simulink model "sampleModel7127"  (R2017a)
settings: Solver=VariableStepAuto  StartTime=0.0  StopTime=10.0  RelTol=1e-3
undefined symbols (not defined in the file or in its folder): DiscIntNeverNeededParam, sigbuilder_block
libraries: simulink x258
(part 1 of 4)
settings Model: Creator=cyfuzz  LastModifiedBy=cyfuzz

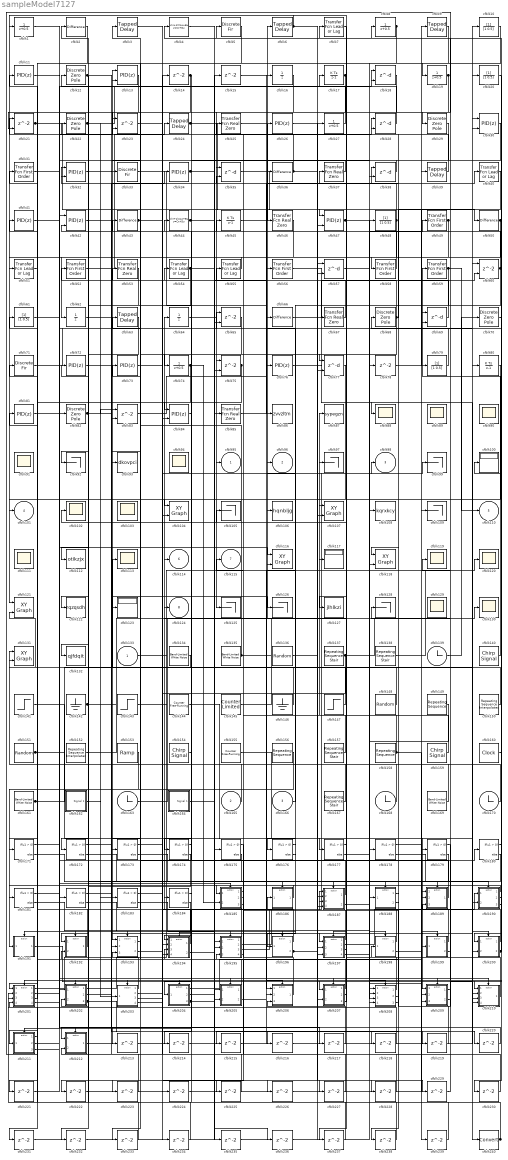
== system sampleModel7127 ==
  cfblk133 : Inport
  cfblk165 : Inport  Port=2
  cfblk166 : Inport  Port=3
  cfblk{1,8,19,27,74} (5 alike) : DiscreteTransferFcn  SampleTime=1
  cfblk{10,20,48,61,79} (5 alike) : DiscreteFilter  SampleTime=1
  cfblk100 : Display
  cfblk{88..91,94,102..103,111,113,119..120,129..130} (13 alike) : Scope
      cfblk103 settings: Floating=on
      cfblk111 settings: Floating=on
      cfblk129 settings: Floating=on
      cfblk89 settings: Floating=on
      cfblk90 settings: Floating=on
      cfblk91 settings: Floating=on
      cfblk94 settings: Floating=on
  cfblk{104,107,116,118,121,131} (6 alike) : simulink/Sinks/XY Graph  xmin=-1  xmax=1  ymin=-1  ymax=1  st=-1
  cfblk{92,97,99,105,109,125..126,128} (8 alike) : Terminator
  cfblk106 : ToWorkspace  VariableName=hqnbljg  SaveFormat=Timeseries  SampleTime=-1
  cfblk108 : ToWorkspace  VariableName=kqrxkcy  SaveFormat=Timeseries  SampleTime=-1
  cfblk{11,26,34,41,72..73,76,81} (8 alike) : simulink/Continuous/PID Controller  Controller=PID  TimeDomain=Discrete-time  SampleTime=1  IntegratorMethod=Forward Euler  FilterMethod=Forward Euler  Form=Parallel  UseFilter=on  ControllerParametersSource=internal  P=1  I=1  D=0  N=100  InitialConditionSource=internal  InitialConditionForIntegrator=0  InitialConditionForFilter=0  ExternalReset=none  LimitOutput=off  UpperSaturationLimit=inf  LowerSaturationLimit=-inf  LinearizeAsGain=off  AntiWindupMode=none  Kb=1  TrackingMode=off  Kt=1  PParamMin=[]  PParamMax=[]  IParamMin=[]  IParamMax=[]  DParamMin=[]  DParamMax=[]  NParamMin=[]  NParamMax=[]  KbParamMin=[]  KbParamMax=[]  KtParamMin=[]  KtParamMax=[]  POutMin=[]  POutMax=[]  IOutMin=[]  IOutMax=[]  DOutMin=[]  DOutMax=[]  NOutMin=[]  NOutMax=[]  KbOutMin=[]  KbOutMax=[]  KtOutMin=[]  KtOutMax=[]  IntegratorOutMin=[]  IntegratorOutMax=[]  FilterOutMin=[]  FilterOutMax=[]  SumOutMin=[]  SumOutMax=[]  SumI1OutMin=[]  SumI1OutMax=[]  SumI2OutMin=[]  SumI2OutMax=[]  SumI3OutMin=[]  SumI3OutMax=[]  SumDOutMin=[]  SumDOutMax=[]  SaturationOutMin=[]  SaturationOutMax=[]  IntegratorContinuousStateAttributes=''  IntegratorStateMustResolveToSignalObject=off  IntegratorRTWStateStorageClass=Auto  FilterContinuousStateAttributes=''  FilterStateMustResolveToSignalObject=off  FilterRTWStateStorageClass=Auto  DifferentiatorICPrevScaledInput=0  DifferentiatorOutMin=[]  DifferentiatorOutMax=[]  InitialConditionSetting=State (most efficient)
  cfblk112 : ToWorkspace  VariableName=otikzjx  SaveFormat=Timeseries  SampleTime=-1
  cfblk117 : Display
  cfblk{12,22,29,68,70,82} (6 alike) : DiscreteZeroPole  Poles=[0 0.5]  Gain=1
  cfblk122 : ToWorkspace  VariableName=rqzqsdh  SaveFormat=Timeseries  SampleTime=-1
  cfblk123 : Display
  cfblk127 : ToWorkspace  VariableName=jlhlkzi  SaveFormat=Timeseries  SampleTime=-1
  cfblk{13,30,32,42,47,84} (6 alike) : simulink/Continuous/PID Controller (2DOF)  Controller=PID  TimeDomain=Discrete-time  SampleTime=1  IntegratorMethod=Forward Euler  FilterMethod=Forward Euler  Form=Parallel  UseFilter=on  ControllerParametersSource=internal  P=1  I=1  D=0  N=100  b=1  c=1  InitialConditionSource=internal  InitialConditionForIntegrator=0  InitialConditionForFilter=0  ExternalReset=none  LimitOutput=off  UpperSaturationLimit=inf  LowerSaturationLimit=-inf  LinearizeAsGain=off  AntiWindupMode=none  Kb=1  TrackingMode=off  Kt=1  PParamMin=[]  PParamMax=[]  IParamMin=[]  IParamMax=[]  DParamMin=[]  DParamMax=[]  NParamMin=[]  NParamMax=[]  bParamMin=[]  bParamMax=[]  cParamMin=[]  cParamMax=[]  KbParamMin=[]  KbParamMax=[]  KtParamMin=[]  KtParamMax=[]  POutMin=[]  POutMax=[]  IOutMin=[]  IOutMax=[]  DOutMin=[]  DOutMax=[]  NOutMin=[]  NOutMax=[]  bOutMin=[]  bOutMax=[]  cOutMin=[]  cOutMax=[]  KbOutMin=[]  KbOutMax=[]  KtOutMin=[]  KtOutMax=[]  IntegratorOutMin=[]  IntegratorOutMax=[]  FilterOutMin=[]  FilterOutMax=[]  SumOutMin=[]  SumOutMax=[]  Sum1OutMin=[]  Sum1OutMax=[]  Sum2OutMin=[]  Sum2OutMax=[]  Sum3OutMin=[]  Sum3OutMax=[]  SumI1OutMin=[]  SumI1OutMax=[]  SumI2OutMin=[]  SumI2OutMax=[]  SumI3OutMin=[]  SumI3OutMax=[]  SumDOutMin=[]  SumDOutMax=[]  SaturationOutMin=[]  SaturationOutMax=[]  IntegratorContinuousStateAttributes=''  IntegratorStateMustResolveToSignalObject=off  IntegratorRTWStateStorageClass=Auto  FilterContinuousStateAttributes=''  FilterStateMustResolveToSignalObject=off  FilterRTWStateStorageClass=Auto  DifferentiatorICPrevScaledInput=0  DifferentiatorOutMin=[]  DifferentiatorOutMax=[]  InitialConditionSetting=State (most efficient)
  cfblk132 : ToWorkspace  VariableName=qjfdqit  SaveFormat=Timeseries  SampleTime=-1
  cfblk{134..135,161,169} (4 alike) : simulink/Sources/Band-Limited White Noise  Cov=[0.1]  Ts=0.1  seed=[23341]
  cfblk136 : RandomNumber  SampleTime=0.1
  cfblk{137..138,157,167} (4 alike) : simulink/Sources/Repeating Sequence Stair  OutValues=[3 1 4 2 1].'  tsamp=-1  OutMin=[]  OutMax=[]  OutDataTypeStr=double  OutputDataTypeScalingMode=double  OutDataType=fixdt(0,8)  ConRadixGroup=Best Precision: Vector-wise  OutScaling=2^-12
  cfblk{139,163,168,170} (4 alike) : Clock
  cfblk{14..15,78,213..239} (30 alike) : Delay  SampleTime=1
  cfblk140 : simulink/Sources/Chirp Signal  f1=0.1  T=100  f2=1
  cfblk141 : Step  After=53  SampleTime=0
  cfblk142 : Ground
  cfblk143 : Step  After=78  SampleTime=0
  cfblk144 : simulink/Sources/Counter Free-Running  NumBits=16  tsamp=-1
  cfblk145 : simulink/Sources/Counter Limited  uplimit=7  tsamp=-1
  cfblk146 : Ground
  cfblk147 : Step  After=42  SampleTime=0
  cfblk148 : RandomNumber  SampleTime=0.1
  cfblk149 : simulink/Sources/Repeating Sequence  rep_seq_t=[0 2]  rep_seq_y=[0 2]
  cfblk150 : simulink/Sources/Repeating Sequence Interpolated  OutValues=[3 1 4 2 1].'  TimeValues=[0 0.1 0.5 0.6 1].'  LookUpMeth=Interpolation-Use End Values  tsamp=0.01  OutMin=[]  OutMax=[]  OutDataTypeStr=double  OutputDataTypeScalingMode=double  OutDataType=fixdt(0,8)  OutScaling=2^-10
  cfblk151 : UniformRandomNumber  SampleTime=0.1
  cfblk152 : simulink/Sources/Repeating Sequence Interpolated  OutValues=[3 1 4 2 1].'  TimeValues=[0 0.1 0.5 0.6 1].'  LookUpMeth=Interpolation-Use End Values  tsamp=0.01  OutMin=[]  OutMax=[]  OutDataTypeStr=double  OutputDataTypeScalingMode=double  OutDataType=fixdt(0,8)  OutScaling=2^-10
  cfblk153 : simulink/Sources/Ramp  slope=1  start=0  X0=0
  cfblk154 : simulink/Sources/Chirp Signal  f1=0.1  T=100  f2=1
  cfblk155 : simulink/Sources/Counter Free-Running  NumBits=16  tsamp=-1
  cfblk156 : simulink/Sources/Repeating Sequence  rep_seq_t=[0 2]  rep_seq_y=[0 2]
  cfblk158 : simulink/Sources/Repeating Sequence  rep_seq_t=[0 2]  rep_seq_y=[0 2]
  cfblk159 : simulink/Sources/Chirp Signal  f1=0.1  T=100  f2=1
  cfblk16 : UnitDelay
  cfblk160 : DigitalClock
  cfblk162 : Subsystem  Tag=STV Subsys  LoadFcn=sigbuilder_block('load');  StartFcn=sigbuilder_block('start');  StopFcn=sigbuilder_block('stop');  ClipboardFcn=sigbuilder_block('clipboard');  mask(Sigbuilder block){tuvar=[0:10]}
      mask help: Simulink:masks:SigbuilderBlock_MD
      mask init:
      | if ~strcmp(get_param(bdroot(gcbh),'SimulationStatus'),'stopped') tuvar = sigbuilder_block('maskInit'); end
      settings: CopyFcn=sigbuilder_block('copy');  DeleteFcn=sigbuilder_block('delete');  ModelCloseFcn=sigbuilder_block('modelClose');  PreSaveFcn=sigbuilder_block('preSave');  PauseFcn=sigbuilder_block('pause');  ContinueFcn=sigbuilder_block('continue');  NameChangeFcn=sigbuilder_block('namechange');  OpenFcn=sigbuilder_block('open',[437.6 199.2 550.4 400 ]);  CloseFcn=sigbuilder_block('close');
      mask Display: plot(0, 0, 100, 100,[2, 2, 32, 32, 2], [68, 8, 8, 68, 68],[32, 2], [38, 38], [32, 19, 2],[53, 60, 44], [32, 17, 17, 2],[16, 16, 31, 31]);txt = getActiveGroup(gcbh);text(2, 100, txt,'verticalAlignment', 'top');
  cfblk164 : Subsystem  Tag=STV Subsys  LoadFcn=sigbuilder_block('load');  StartFcn=sigbuilder_block('start');  StopFcn=sigbuilder_block('stop');  ClipboardFcn=sigbuilder_block('clipboard');  mask(Sigbuilder block){tuvar=[0:10]}
      mask help: Simulink:masks:SigbuilderBlock_MD
      mask init:
      | if ~strcmp(get_param(bdroot(gcbh),'SimulationStatus'),'stopped') tuvar = sigbuilder_block('maskInit'); end
      settings: CopyFcn=sigbuilder_block('copy');  DeleteFcn=sigbuilder_block('delete');  ModelCloseFcn=sigbuilder_block('modelClose');  PreSaveFcn=sigbuilder_block('preSave');  PauseFcn=sigbuilder_block('pause');  ContinueFcn=sigbuilder_block('continue');  NameChangeFcn=sigbuilder_block('namechange');  OpenFcn=sigbuilder_block('open',[437.6 199.2 550.4 400 ]);  CloseFcn=sigbuilder_block('close');
      mask Display: plot(0, 0, 100, 100,[2, 2, 32, 32, 2], [68, 8, 8, 68, 68],[32, 2], [38, 38], [32, 19, 2],[53, 60, 44], [32, 17, 17, 2],[16, 16, 31, 31]);txt = getActiveGroup(gcbh);text(2, 100, txt,'verticalAlignment', 'top');
  cfblk17 : DiscreteIntegrator  InitialConditionSetting=State (most efficient)  ICPrevOutput=DiscIntNeverNeededParam  ICPrevScaledInput=DiscIntNeverNeededParam
  cfblk{171..184} (14 alike) : If  SampleTime=1
  cfblk{18,28,35,38,57,69,77} (7 alike) : Delay  DelayLengthSource=Input port  SampleTime=1
      settings: InputPortMap=u0,p1
  cfblk185 : Subsystem  TreatAsAtomicUnit=on
  cfblk186 : Subsystem  TreatAsAtomicUnit=on
  cfblk187 : Subsystem  TreatAsAtomicUnit=on
  cfblk188 : Subsystem  TreatAsAtomicUnit=on
  cfblk189 : Subsystem  TreatAsAtomicUnit=on
  cfblk190 : Subsystem  TreatAsAtomicUnit=on
  cfblk191 : Subsystem  TreatAsAtomicUnit=on
  cfblk192 : Subsystem  TreatAsAtomicUnit=on
  cfblk193 : Subsystem  TreatAsAtomicUnit=on
  cfblk194 : Subsystem  TreatAsAtomicUnit=on
  cfblk195 : Subsystem  TreatAsAtomicUnit=on
  cfblk196 : Subsystem  TreatAsAtomicUnit=on
  cfblk197 : Subsystem  TreatAsAtomicUnit=on
  cfblk198 : Subsystem  TreatAsAtomicUnit=on
  cfblk199 : Subsystem  TreatAsAtomicUnit=on
  cfblk{2,36,43,50,66} (5 alike) : simulink/Discrete/Difference  ICPrevInput=0.0  OutMin=[]  OutMax=[]  OutDataTypeStr=Inherit: Inherit via back propagation  OutDataType=fixdt(1, 16)  OutScaling=2^-10  DoSatur=off
  cfblk200 : Subsystem  TreatAsAtomicUnit=on
  cfblk201 : Subsystem  TreatAsAtomicUnit=on
  cfblk202 : Subsystem  TreatAsAtomicUnit=on
  cfblk203 : Subsystem  TreatAsAtomicUnit=on
  cfblk204 : Subsystem  TreatAsAtomicUnit=on
  cfblk205 : Subsystem  TreatAsAtomicUnit=on
  cfblk206 : Subsystem  TreatAsAtomicUnit=on
  cfblk207 : Subsystem  TreatAsAtomicUnit=on
  cfblk208 : Subsystem  TreatAsAtomicUnit=on
  cfblk209 : Subsystem  TreatAsAtomicUnit=on
  cfblk{21,23,60,65,75,83} (6 alike) : Delay  ShowEnablePort=on  SampleTime=1
      settings: InputPortMap=u0,e6
  cfblk210 : Subsystem  TreatAsAtomicUnit=on
  cfblk211 : Subsystem  TreatAsAtomicUnit=on
  cfblk212 : Subsystem  TreatAsAtomicUnit=on
  cfblk{3,6,9,24,39,63} (6 alike) : simulink/Discrete/Tapped Delay  vinit=0.0  samptime=-1  NumDelays=1  DelayOrder=Oldest  includeCurrent=off
  cfblk240 : DataTypeConversion
  cfblk{25,37,46,53,67,85} (6 alike) : simulink/Discrete/Transfer Fcn Real Zero  ZeroZ=0.75  ICPrevInput=0.0  DoSatur=off
      settings: SourceProductName=Simulink  SourceProductBaseCode=SL
  cfblk{31,49,52,56,58..59} (6 alike) : simulink/Discrete/Transfer Fcn First Order  PoleZ=0.95  ICPrevOutput=0.0  DoSatur=off
      settings: SourceProductName=Simulink
  cfblk33 : DiscreteFir  SampleTime=1
  cfblk4 : DiscreteStateSpace
  cfblk{7,40,51,54..55} (5 alike) : simulink/Discrete/Transfer Fcn Lead or Lag  PoleZ=0.95  ZeroZ=0.75  ICPrevOutput=0.0  ICPrevInput=0.0  DoSatur=off
      settings: SourceProductName=Simulink  SourceProductBaseCode=SL
  cfblk44 : DiscreteStateSpace
  cfblk45 : DiscreteIntegrator  InitialConditionSetting=State (most efficient)  ICPrevOutput=DiscIntNeverNeededParam  ICPrevScaledInput=DiscIntNeverNeededParam
  cfblk5 : DiscreteFir  SampleTime=1
  cfblk62 : UnitDelay
  cfblk64 : UnitDelay
  cfblk71 : DiscreteFir  SampleTime=1
  cfblk80 : DiscreteIntegrator  InitialConditionSetting=State (most efficient)  ICPrevOutput=DiscIntNeverNeededParam  ICPrevScaledInput=DiscIntNeverNeededParam
  cfblk86 : ToWorkspace  VariableName=zvvzltm  SaveFormat=Timeseries  SampleTime=-1
  cfblk87 : ToWorkspace  VariableName=sypegzn  SaveFormat=Timeseries  SampleTime=-1
  cfblk93 : ToWorkspace  VariableName=dkovpci  SaveFormat=Timeseries  SampleTime=-1
  cfblk95 : Outport
  cfblk96 : Outport  Port=2
  cfblk98 : Outport  Port=3
  cfblk101 : Outport  Port=4
  cfblk110 : Outport  Port=5
  cfblk114 : Outport  Port=6
  cfblk115 : Outport  Port=7
  cfblk124 : Outport  Port=8
  wires:
  cfblk139/1 -> cfblk70/1
  cfblk17/1 -> cfblk125/1, cfblk47/2
  cfblk162/1(Signal 1) -> cfblk203/1(cfblk1)
  cfblk13/1 -> cfblk193/1(cfblk1)
  cfblk49/1 -> cfblk62/1, cfblk238/1
  cfblk144/1 -> cfblk209/1(cfblk1)
  cfblk157/1 -> cfblk87/1
  cfblk156/1 -> cfblk191/1(cfblk1)
  cfblk143/1 -> cfblk6/1
  cfblk207/1(cfblk2) -> cfblk63/1
  cfblk52/1 -> cfblk24/1
  cfblk20/1 -> cfblk186/1(cfblk1)
  cfblk81/1 -> cfblk82/1
  cfblk28/1 -> cfblk121/1
  cfblk148/1 -> cfblk113/1
  cfblk187/1(cfblk2) -> cfblk73/1
  cfblk50/1 -> cfblk210/1(cfblk1), cfblk118/1
  cfblk64/1 -> cfblk95/1
  cfblk6/1 -> cfblk1/1, cfblk210/3(cfblk16)
  cfblk202/1(cfblk2) -> cfblk120/1
  cfblk55/1 -> cfblk51/1
  cfblk195/1(cfblk2) -> cfblk52/1
  cfblk72/1 -> cfblk126/1
  cfblk167/1 -> cfblk131/1
  cfblk196/1(cfblk2) -> cfblk64/1
  cfblk166/1 -> cfblk66/1
  cfblk204/1(cfblk2) -> cfblk39/1
  cfblk201/1(cfblk2) -> cfblk123/1
  cfblk33/1 -> cfblk86/1
  cfblk199/1(cfblk2) -> cfblk5/1
  cfblk16/1 -> cfblk173/1
  cfblk53/1 -> cfblk192/1(cfblk1)
  cfblk24/1 -> cfblk47/1, cfblk200/2(cfblk7)
  cfblk2/1 -> cfblk211/1(cfblk1)
  cfblk27/1 -> cfblk12/1
  cfblk142/1 -> cfblk85/1, cfblk108/1
  cfblk140/1 -> cfblk59/1
  cfblk195/2(cfblk15) -> cfblk98/1
  cfblk133/1 -> cfblk97/1
  cfblk63/1 -> cfblk122/1
  cfblk190/1(cfblk2) -> cfblk181/1
  cfblk191/1(cfblk2) -> cfblk207/1(cfblk1)
  cfblk147/1 -> cfblk43/1
  cfblk36/1 -> cfblk13/1, cfblk199/1(cfblk1)
  cfblk41/1 -> cfblk182/1
  cfblk169/1 -> cfblk71/1
  cfblk195/3(cfblk16) -> cfblk9/1
  cfblk160/1 -> cfblk100/1
  cfblk209/1(cfblk2) -> cfblk119/1
  cfblk68/1 -> cfblk75/1, cfblk28/1, cfblk127/1, cfblk32/2
  cfblk199/2(cfblk10) -> cfblk128/1
  cfblk83/1 -> cfblk76/1
  cfblk51/1 -> cfblk171/1
  cfblk25/1 -> cfblk46/1
  cfblk195/4(cfblk17) -> cfblk105/1
  cfblk1/1 -> cfblk116/1
  cfblk164/1(Signal 1) -> cfblk15/1
  cfblk208/1(cfblk2) -> cfblk187/1(cfblk1)
  cfblk159/1 -> cfblk55/1
  cfblk54/1 -> cfblk179/1, cfblk83/2
  cfblk135/1 -> cfblk53/1, cfblk107/2
  cfblk82/1 -> cfblk83/1, cfblk220/1
  cfblk22/1 -> cfblk16/1, cfblk183/1
  cfblk21/1 -> cfblk50/1, cfblk217/1
  cfblk75/1 -> cfblk84/1, cfblk92/1
  cfblk197/1(cfblk2) -> cfblk115/1
  cfblk192/1(cfblk2) -> cfblk61/1
  cfblk193/1(cfblk2) -> cfblk3/1
  cfblk161/1 -> cfblk109/1, cfblk77/2
  cfblk165/1 -> cfblk31/1
  cfblk145/1 -> cfblk80/1
  cfblk85/1 -> cfblk40/1
  cfblk151/1 -> cfblk27/1, cfblk20/1
  cfblk152/1 -> cfblk114/1
  cfblk48/1 -> cfblk37/1, cfblk205/2(cfblk8), cfblk237/1
  cfblk47/1 -> cfblk178/1, cfblk209/3(cfblk13)
  cfblk212/1(cfblk2) -> cfblk14/1
  cfblk74/1 -> cfblk185/2(cfblk14), cfblk221/1
  cfblk207/2(cfblk15) -> cfblk106/1
  cfblk35/1 -> cfblk79/1
  cfblk34/1 -> cfblk226/1, cfblk227/1
  cfblk153/1 -> cfblk201/1(cfblk1)
  cfblk12/1 -> cfblk132/1, cfblk195/2(cfblk13)
  cfblk39/1 -> cfblk13/2
  cfblk202/2(cfblk12) -> cfblk34/1
  cfblk158/1 -> cfblk209/2(cfblk12), cfblk35/2
  cfblk194/1(cfblk2) -> cfblk81/1
  cfblk38/1 -> cfblk35/1
  cfblk80/1 -> cfblk101/1
  cfblk43/1 -> cfblk93/1, cfblk210/2(cfblk15)
  cfblk58/1 -> cfblk45/1
  cfblk197/2(cfblk15) -> cfblk190/1(cfblk1)
  cfblk137/1 -> cfblk17/1, cfblk194/4(cfblk8), cfblk130/1
  cfblk46/1 -> cfblk112/1
  cfblk168/1 -> cfblk96/1
  cfblk207/3(cfblk16) -> cfblk124/1
  cfblk45/1 -> cfblk177/1
  cfblk136/1 -> cfblk57/1
  cfblk202/3(cfblk13) -> cfblk69/1, cfblk234/1
  cfblk79/1 -> cfblk68/1
  cfblk30/1 -> cfblk174/1
  cfblk205/1(cfblk2) -> cfblk11/1
  cfblk56/1 -> cfblk190/2(cfblk13)
  cfblk200/1(cfblk2) -> cfblk26/1
  cfblk44/1 -> cfblk194/1(cfblk1), cfblk236/1
  cfblk210/1(cfblk2) -> cfblk32/1
  cfblk5/1 -> cfblk23/1
  cfblk77/1 -> cfblk104/1
  cfblk197/3(cfblk16) -> cfblk102/1
  cfblk15/1 -> cfblk206/1(cfblk1)
  cfblk138/1 -> cfblk10/1
  cfblk9/1 -> cfblk19/1
  cfblk62/1 -> cfblk197/1(cfblk1)
  cfblk150/1 -> cfblk116/2
  cfblk67/1 -> cfblk54/1
  cfblk211/1(cfblk2) -> cfblk29/1
  cfblk193/2(cfblk17) -> cfblk104/2
  cfblk146/1 -> cfblk121/2
  cfblk154/1 -> cfblk204/1(cfblk1)
  cfblk198/1(cfblk2) -> cfblk4/1
  cfblk205/2(cfblk9) -> cfblk117/1
  cfblk134/1 -> cfblk131/2
  cfblk190/2(cfblk14) -> cfblk42/2
  cfblk4/1 -> cfblk205/1(cfblk1)
  cfblk18/1 -> cfblk172/1
  cfblk7/1 -> cfblk77/1
  cfblk197/4(cfblk17) -> cfblk48/1
  cfblk14/1 -> cfblk74/1, cfblk84/2, cfblk21/2
  cfblk19/1 -> cfblk65/2, cfblk232/1
  cfblk57/1 -> cfblk78/1
  cfblk187/2(cfblk16) -> cfblk49/1
  cfblk40/1 -> cfblk58/1
  cfblk31/1 -> cfblk18/1
  cfblk204/2(cfblk9) -> cfblk56/1
  cfblk60/1 -> cfblk196/1(cfblk1), cfblk25/1
  cfblk73/1 -> cfblk197/3(cfblk14)
  cfblk10/1 -> cfblk33/1
  cfblk186/1(cfblk2) -> cfblk185/1(cfblk1)
  cfblk59/1 -> cfblk176/1, cfblk110/1
  cfblk69/1 -> cfblk38/1
  cfblk200/2(cfblk8) -> cfblk7/1, cfblk230/1
  cfblk211/2(cfblk14) -> cfblk180/1
  cfblk163/1 -> cfblk75/2
  cfblk76/1 -> cfblk88/1
  cfblk149/1 -> cfblk208/2(cfblk13)
  cfblk71/1 -> cfblk30/1
  cfblk66/1 -> cfblk30/2
  cfblk141/1 -> cfblk208/3(cfblk14)
  cfblk78/1 -> cfblk60/2
  cfblk190/3(cfblk15) -> cfblk69/2
  cfblk208/2(cfblk16) -> cfblk198/1(cfblk1)
  cfblk206/1(cfblk2) -> cfblk21/1
  cfblk61/1 -> cfblk202/1(cfblk1)
  cfblk196/2(cfblk10) -> cfblk67/1, cfblk210/4(cfblk17)
  cfblk204/3(cfblk10) -> cfblk192/2(cfblk8), cfblk28/2
  cfblk209/2(cfblk14) -> cfblk8/1
  cfblk211/3(cfblk15) -> cfblk23/2
  cfblk11/1 -> cfblk38/2
  cfblk29/1 -> cfblk57/2
  cfblk189/1(cfblk2) -> cfblk44/1
  cfblk208/3(cfblk17) -> cfblk194/3(cfblk7)
  cfblk155/1 -> cfblk240/1
  cfblk170/1 -> cfblk107/1
  cfblk201/3(cfblk12) -> cfblk41/1
  cfblk8/1 -> cfblk118/2, cfblk231/1
  cfblk70/1 -> cfblk200/1(cfblk1)
  cfblk201/4(cfblk13) -> cfblk65/1
  cfblk203/1(cfblk2) -> cfblk193/3(cfblk16)
  cfblk37/1 -> cfblk36/1
  cfblk203/2(cfblk8) -> cfblk187/3(cfblk14)
  cfblk203/3(cfblk9) -> cfblk99/1
  cfblk203/4(cfblk10) -> cfblk18/2
  cfblk171/1 -> cfblk185/Action
  cfblk171/2 -> cfblk186/Action
  cfblk172/1 -> cfblk187/Action
  cfblk172/2 -> cfblk188/Action
  cfblk173/1 -> cfblk189/Action
  cfblk173/2 -> cfblk190/Action
  cfblk174/1 -> cfblk191/Action
  cfblk174/2 -> cfblk192/Action
  cfblk175/1 -> cfblk193/Action
  cfblk175/2 -> cfblk194/Action
  cfblk176/1 -> cfblk195/Action
  cfblk176/2 -> cfblk196/Action
  cfblk177/1 -> cfblk197/Action
  cfblk177/2 -> cfblk198/Action
  cfblk178/1 -> cfblk199/Action
  cfblk178/2 -> cfblk200/Action
  cfblk179/1 -> cfblk201/Action
  cfblk179/2 -> cfblk202/Action
  cfblk180/1 -> cfblk203/Action
  cfblk180/2 -> cfblk204/Action
  cfblk181/1 -> cfblk205/Action
  cfblk181/2 -> cfblk206/Action
  cfblk182/1 -> cfblk207/Action
  cfblk182/2 -> cfblk208/Action
  cfblk183/1 -> cfblk209/Action
  cfblk183/2 -> cfblk210/Action
  cfblk184/1 -> cfblk211/Action
  cfblk184/2 -> cfblk212/Action
  cfblk201/2(cfblk11) -> cfblk213/1
  cfblk213/1 -> cfblk60/1
  cfblk84/1 -> cfblk214/1
  cfblk214/1 -> cfblk188/1(cfblk1)
  cfblk188/1(cfblk2) -> cfblk215/1
  cfblk215/1 -> cfblk206/2(cfblk16)
  cfblk32/1 -> cfblk216/1
  cfblk216/1 -> cfblk208/1(cfblk1)
  cfblk217/1 -> cfblk206/3(cfblk17)
  cfblk188/2(cfblk11) -> cfblk218/1
  cfblk218/1 -> cfblk201/3(cfblk9)
  cfblk42/1 -> cfblk219/1
  cfblk219/1 -> cfblk189/1(cfblk1)
  cfblk220/1 -> cfblk212/1(cfblk1)
  cfblk221/1 -> cfblk42/1
  cfblk185/1(cfblk2) -> cfblk222/1
  cfblk222/1 -> cfblk207/2(cfblk14)
  cfblk185/2(cfblk15) -> cfblk223/1
  cfblk223/1 -> cfblk193/2(cfblk15)
  cfblk3/1 -> cfblk224/1
  cfblk224/1 -> cfblk189/2(cfblk7)
  cfblk185/3(cfblk16) -> cfblk225/1
  cfblk225/1 -> cfblk202/2(cfblk11)
  cfblk226/1 -> cfblk187/2(cfblk13)
  cfblk227/1 -> cfblk195/3(cfblk14)
  cfblk23/1 -> cfblk228/1
  cfblk228/1 -> cfblk2/1
  cfblk26/1 -> cfblk229/1
  cfblk229/1 -> cfblk189/3(cfblk8)
  cfblk230/1 -> cfblk194/2(cfblk6)
  cfblk231/1 -> cfblk175/1
  cfblk232/1 -> cfblk197/2(cfblk13)
  cfblk65/1 -> cfblk233/1
  cfblk233/1 -> cfblk212/2(cfblk9)
  cfblk234/1 -> cfblk201/4(cfblk10)
  cfblk194/2(cfblk9) -> cfblk235/1
  cfblk235/1 -> cfblk208/4(cfblk15)
  cfblk236/1 -> cfblk187/4(cfblk15)
  cfblk237/1 -> cfblk195/1(cfblk1)
  cfblk238/1 -> cfblk184/1
  cfblk198/2(cfblk10) -> cfblk239/1
  cfblk239/1 -> cfblk201/2(cfblk8)
  cfblk240/1 -> cfblk72/1, cfblk22/1

== system sampleModel7127/cfblk162 ==
  Demux : Demux  Tag=STV Demux  Outputs=1
  FromWs : FromWorkspace  Tag=STV FromWs  VariableName=tuvar  SampleTime=0
      SigBuilderData=|
      | common.afterFinalStr = 'Extrapolate'
      | common.sampleTime = 0
      | dataSet.timeRange = [0 10]
      | dataSet.name = 'Group 1'
      | sbobj.Groups.Name = 'Group 1'
      | sbobj.Groups.Signals.Name = 'Signal 1'
      | sbobj.Groups.Signals.XData = [0 4 4 6 6 10]
      | sbobj.Groups.Signals.YData = [0 0 1 1 0 0]
  Signal 1 : Outport  Tag=STV Outport
  wires:
  Demux/1 -> Signal 1/1
  FromWs/1 -> Demux/1

== system sampleModel7127/cfblk164 ==
  Demux : Demux  Tag=STV Demux  Outputs=1
  FromWs : FromWorkspace  Tag=STV FromWs  VariableName=tuvar  SampleTime=0
      SigBuilderData=|
      | common.afterFinalStr = 'Extrapolate'
      | common.sampleTime = 0
      | dataSet.timeRange = [0 10]
      | dataSet.name = 'Group 1'
      | sbobj.Groups.Name = 'Group 1'
      | sbobj.Groups.Signals.Name = 'Signal 1'
      | sbobj.Groups.Signals.XData = [0 4 4 6 6 10]
      | sbobj.Groups.Signals.YData = [0 0 1 1 0 0]
  Signal 1 : Outport  Tag=STV Outport
  wires:
  Demux/1 -> Signal 1/1
  FromWs/1 -> Demux/1

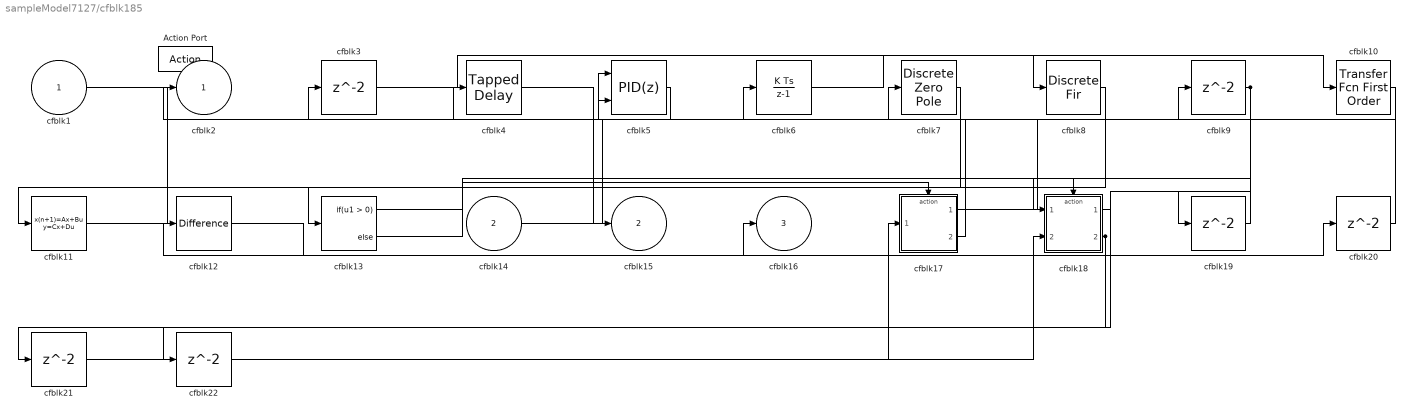
== system sampleModel7127/cfblk185 ==
  cfblk1 : Inport
  cfblk14 : Inport  Port=2
  Action Port : ActionPort  ActionType=then
  cfblk10 : simulink/Discrete/Transfer Fcn First Order  PoleZ=0.95  ICPrevOutput=0.0  DoSatur=off
      settings: SourceProductName=Simulink
  cfblk11 : DiscreteStateSpace  SampleTime=-1
  cfblk12 : simulink/Discrete/Difference  ICPrevInput=0.0  OutMin=[]  OutMax=[]  OutDataTypeStr=Inherit: Inherit via back propagation  OutDataType=fixdt(1, 16)  OutScaling=2^-10  DoSatur=off
  cfblk13 : If  SampleTime=1
  cfblk17 : Subsystem  TreatAsAtomicUnit=on
  cfblk18 : Subsystem  TreatAsAtomicUnit=on
  cfblk{3,9,19..22} (6 alike) : Delay
  cfblk4 : simulink/Discrete/Tapped Delay  vinit=0.0  samptime=-1  NumDelays=1  DelayOrder=Oldest  includeCurrent=off
  cfblk5 : simulink/Continuous/PID Controller (2DOF)  Controller=PID  TimeDomain=Discrete-time  SampleTime=-1  IntegratorMethod=Forward Euler  FilterMethod=Forward Euler  Form=Parallel  UseFilter=on  ControllerParametersSource=internal  P=1  I=1  D=0  N=100  b=1  c=1  InitialConditionSource=internal  InitialConditionForIntegrator=0  InitialConditionForFilter=0  ExternalReset=none  LimitOutput=off  UpperSaturationLimit=inf  LowerSaturationLimit=-inf  LinearizeAsGain=off  AntiWindupMode=none  Kb=1  TrackingMode=off  Kt=1  PParamMin=[]  PParamMax=[]  IParamMin=[]  IParamMax=[]  DParamMin=[]  DParamMax=[]  NParamMin=[]  NParamMax=[]  bParamMin=[]  bParamMax=[]  cParamMin=[]  cParamMax=[]  KbParamMin=[]  KbParamMax=[]  KtParamMin=[]  KtParamMax=[]  POutMin=[]  POutMax=[]  IOutMin=[]  IOutMax=[]  DOutMin=[]  DOutMax=[]  NOutMin=[]  NOutMax=[]  bOutMin=[]  bOutMax=[]  cOutMin=[]  cOutMax=[]  KbOutMin=[]  KbOutMax=[]  KtOutMin=[]  KtOutMax=[]  IntegratorOutMin=[]  IntegratorOutMax=[]  FilterOutMin=[]  FilterOutMax=[]  SumOutMin=[]  SumOutMax=[]  Sum1OutMin=[]  Sum1OutMax=[]  Sum2OutMin=[]  Sum2OutMax=[]  Sum3OutMin=[]  Sum3OutMax=[]  SumI1OutMin=[]  SumI1OutMax=[]  SumI2OutMin=[]  SumI2OutMax=[]  SumI3OutMin=[]  SumI3OutMax=[]  SumDOutMin=[]  SumDOutMax=[]  SaturationOutMin=[]  SaturationOutMax=[]  IntegratorContinuousStateAttributes=''  IntegratorStateMustResolveToSignalObject=off  IntegratorRTWStateStorageClass=Auto  FilterContinuousStateAttributes=''  FilterStateMustResolveToSignalObject=off  FilterRTWStateStorageClass=Auto  DifferentiatorICPrevScaledInput=0  DifferentiatorOutMin=[]  DifferentiatorOutMax=[]  InitialConditionSetting=State (most efficient)
  cfblk6 : DiscreteIntegrator  InitialConditionSetting=State (most efficient)  SampleTime=-1  ICPrevOutput=DiscIntNeverNeededParam  ICPrevScaledInput=DiscIntNeverNeededParam
  cfblk7 : DiscreteZeroPole  Poles=[0 0.5]  Gain=1  SampleTime=-1
  cfblk8 : DiscreteFir
  cfblk2 : Outport
  cfblk15 : Outport  Port=2
  cfblk16 : Outport  Port=3
  wires:
  cfblk7/1 -> cfblk11/1
  cfblk3/1 -> cfblk10/1
  cfblk17/1(cfblk2) -> cfblk9/1
  cfblk17/2(cfblk8) -> cfblk4/1
  cfblk11/1 -> cfblk3/1
  cfblk8/1 -> cfblk13/1
  cfblk1/1 -> cfblk5/1
  cfblk14/1 -> cfblk7/1
  cfblk6/1 -> cfblk8/1
  cfblk5/1 -> cfblk2/1
  cfblk10/1 -> cfblk5/2
  cfblk4/1 -> cfblk15/1
  cfblk9/1 -> cfblk19/1, cfblk22/1
  cfblk18/1(cfblk2) -> cfblk12/1
  cfblk18/2(cfblk10) -> cfblk16/1, cfblk21/1
  cfblk13/1 -> cfblk17/Action
  cfblk13/2 -> cfblk18/Action
  cfblk19/1 -> cfblk18/1(cfblk1)
  cfblk12/1 -> cfblk20/1
  cfblk20/1 -> cfblk6/1
  cfblk21/1 -> cfblk17/1(cfblk1)
  cfblk22/1 -> cfblk18/2(cfblk9)

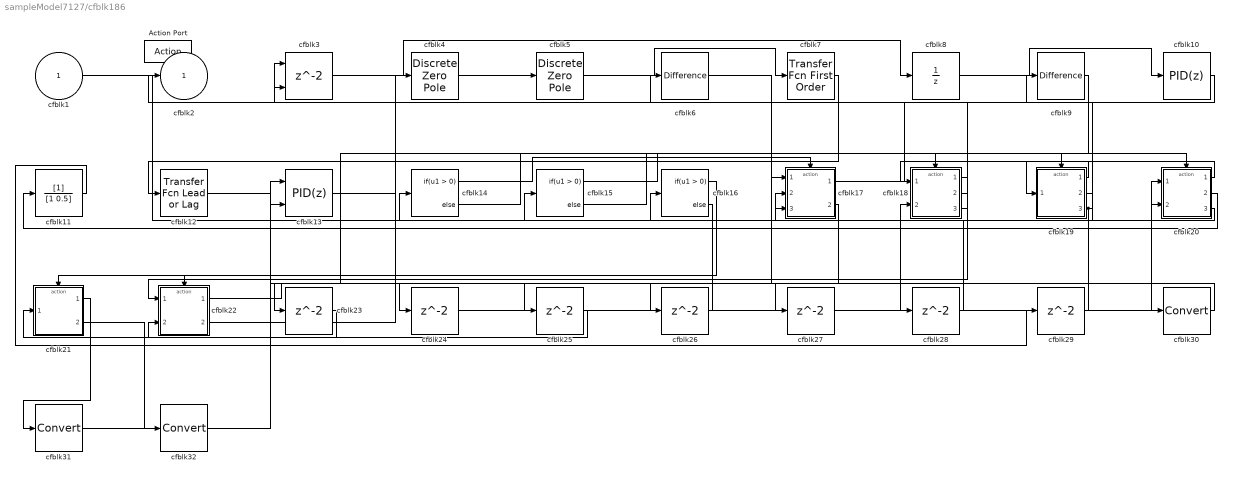
== system sampleModel7127/cfblk186 ==
  cfblk1 : Inport
  Action Port : ActionPort  ActionType=else
  cfblk10 : simulink/Continuous/PID Controller  Controller=PID  TimeDomain=Discrete-time  SampleTime=-1  IntegratorMethod=Forward Euler  FilterMethod=Forward Euler  Form=Parallel  UseFilter=on  ControllerParametersSource=internal  P=1  I=1  D=0  N=100  InitialConditionSource=internal  InitialConditionForIntegrator=0  InitialConditionForFilter=0  ExternalReset=none  LimitOutput=off  UpperSaturationLimit=inf  LowerSaturationLimit=-inf  LinearizeAsGain=off  AntiWindupMode=none  Kb=1  TrackingMode=off  Kt=1  PParamMin=[]  PParamMax=[]  IParamMin=[]  IParamMax=[]  DParamMin=[]  DParamMax=[]  NParamMin=[]  NParamMax=[]  KbParamMin=[]  KbParamMax=[]  KtParamMin=[]  KtParamMax=[]  POutMin=[]  POutMax=[]  IOutMin=[]  IOutMax=[]  DOutMin=[]  DOutMax=[]  NOutMin=[]  NOutMax=[]  KbOutMin=[]  KbOutMax=[]  KtOutMin=[]  KtOutMax=[]  IntegratorOutMin=[]  IntegratorOutMax=[]  FilterOutMin=[]  FilterOutMax=[]  SumOutMin=[]  SumOutMax=[]  SumI1OutMin=[]  SumI1OutMax=[]  SumI2OutMin=[]  SumI2OutMax=[]  SumI3OutMin=[]  SumI3OutMax=[]  SumDOutMin=[]  SumDOutMax=[]  SaturationOutMin=[]  SaturationOutMax=[]  IntegratorContinuousStateAttributes=''  IntegratorStateMustResolveToSignalObject=off  IntegratorRTWStateStorageClass=Auto  FilterContinuousStateAttributes=''  FilterStateMustResolveToSignalObject=off  FilterRTWStateStorageClass=Auto  DifferentiatorICPrevScaledInput=0  DifferentiatorOutMin=[]  DifferentiatorOutMax=[]  InitialConditionSetting=State (most efficient)
  cfblk11 : DiscreteFilter
  cfblk12 : simulink/Discrete/Transfer Fcn Lead or Lag  PoleZ=0.95  ZeroZ=0.75  ICPrevOutput=0.0  ICPrevInput=0.0  DoSatur=off
      settings: SourceProductName=Simulink  SourceProductBaseCode=SL
  cfblk13 : simulink/Continuous/PID Controller (2DOF)  Controller=PID  TimeDomain=Discrete-time  SampleTime=-1  IntegratorMethod=Forward Euler  FilterMethod=Forward Euler  Form=Parallel  UseFilter=on  ControllerParametersSource=internal  P=1  I=1  D=0  N=100  b=1  c=1  InitialConditionSource=internal  InitialConditionForIntegrator=0  InitialConditionForFilter=0  ExternalReset=none  LimitOutput=off  UpperSaturationLimit=inf  LowerSaturationLimit=-inf  LinearizeAsGain=off  AntiWindupMode=none  Kb=1  TrackingMode=off  Kt=1  PParamMin=[]  PParamMax=[]  IParamMin=[]  IParamMax=[]  DParamMin=[]  DParamMax=[]  NParamMin=[]  NParamMax=[]  bParamMin=[]  bParamMax=[]  cParamMin=[]  cParamMax=[]  KbParamMin=[]  KbParamMax=[]  KtParamMin=[]  KtParamMax=[]  POutMin=[]  POutMax=[]  IOutMin=[]  IOutMax=[]  DOutMin=[]  DOutMax=[]  NOutMin=[]  NOutMax=[]  bOutMin=[]  bOutMax=[]  cOutMin=[]  cOutMax=[]  KbOutMin=[]  KbOutMax=[]  KtOutMin=[]  KtOutMax=[]  IntegratorOutMin=[]  IntegratorOutMax=[]  FilterOutMin=[]  FilterOutMax=[]  SumOutMin=[]  SumOutMax=[]  Sum1OutMin=[]  Sum1OutMax=[]  Sum2OutMin=[]  Sum2OutMax=[]  Sum3OutMin=[]  Sum3OutMax=[]  SumI1OutMin=[]  SumI1OutMax=[]  SumI2OutMin=[]  SumI2OutMax=[]  SumI3OutMin=[]  SumI3OutMax=[]  SumDOutMin=[]  SumDOutMax=[]  SaturationOutMin=[]  SaturationOutMax=[]  IntegratorContinuousStateAttributes=''  IntegratorStateMustResolveToSignalObject=off  IntegratorRTWStateStorageClass=Auto  FilterContinuousStateAttributes=''  FilterStateMustResolveToSignalObject=off  FilterRTWStateStorageClass=Auto  DifferentiatorICPrevScaledInput=0  DifferentiatorOutMin=[]  DifferentiatorOutMax=[]  InitialConditionSetting=State (most efficient)
  cfblk14 : If  SampleTime=1
  cfblk15 : If  SampleTime=1
  cfblk16 : If  SampleTime=1
  cfblk17 : Subsystem  TreatAsAtomicUnit=on
  cfblk18 : Subsystem  TreatAsAtomicUnit=on
  cfblk19 : Subsystem  TreatAsAtomicUnit=on
  cfblk20 : Subsystem  TreatAsAtomicUnit=on
  cfblk21 : Subsystem  TreatAsAtomicUnit=on
  cfblk22 : Subsystem  TreatAsAtomicUnit=on
  cfblk{23..29} (7 alike) : Delay
  cfblk3 : Delay  ShowEnablePort=on
      settings: InputPortMap=u0,e6
  cfblk30 : DataTypeConversion
  cfblk31 : DataTypeConversion
  cfblk32 : DataTypeConversion
  cfblk4 : DiscreteZeroPole  Poles=[0 0.5]  Gain=1  SampleTime=-1
  cfblk5 : DiscreteZeroPole  Poles=[0 0.5]  Gain=1  SampleTime=-1
  cfblk6 : simulink/Discrete/Difference  ICPrevInput=0.0  OutMin=[]  OutMax=[]  OutDataTypeStr=Inherit: Inherit via back propagation  OutDataType=fixdt(1, 16)  OutScaling=2^-10  DoSatur=off
  cfblk7 : simulink/Discrete/Transfer Fcn First Order  PoleZ=0.95  ICPrevOutput=0.0  DoSatur=off
      settings: SourceProductName=Simulink
  cfblk8 : UnitDelay  SampleTime=-1
  cfblk9 : simulink/Discrete/Difference  ICPrevInput=0.0  OutMin=[]  OutMax=[]  OutDataTypeStr=Inherit: Inherit via back propagation  OutDataType=fixdt(1, 16)  OutScaling=2^-10  DoSatur=off
  cfblk2 : Outport
  wires:
  cfblk5/1 -> cfblk7/1
  cfblk8/1 -> cfblk10/1
  cfblk20/1(cfblk2) -> cfblk19/1(cfblk1)
  cfblk1/1 -> cfblk20/1(cfblk1)
  cfblk20/2(cfblk15) -> cfblk11/1
  cfblk20/3(cfblk16) -> cfblk16/1
  cfblk4/1 -> cfblk5/1
  cfblk10/1 -> cfblk6/1
  cfblk3/1 -> cfblk8/1
  cfblk18/1(cfblk2) -> cfblk22/1(cfblk1)
  cfblk7/1 -> cfblk12/1
  cfblk17/1(cfblk2) -> cfblk9/1
  cfblk19/1(cfblk2) -> cfblk18/1(cfblk1)
  cfblk22/2(cfblk16) -> cfblk4/1
  cfblk18/2(cfblk10) -> cfblk3/1
  cfblk18/3(cfblk11) -> cfblk3/2
  cfblk19/2(cfblk10) -> cfblk17/2(cfblk13)
  cfblk19/3(cfblk11) -> cfblk2/1, cfblk17/3(cfblk14)
  cfblk14/1 -> cfblk17/Action
  cfblk14/2 -> cfblk18/Action
  cfblk15/1 -> cfblk19/Action
  cfblk15/2 -> cfblk20/Action
  cfblk16/1 -> cfblk21/Action
  cfblk16/2 -> cfblk22/Action
  cfblk9/1 -> cfblk23/1
  cfblk23/1 -> cfblk21/1(cfblk1)
  cfblk24/1 -> cfblk20/2(cfblk14)
  cfblk17/2(cfblk15) -> cfblk25/1
  cfblk25/1 -> cfblk22/2(cfblk15)
  cfblk22/1(cfblk2) -> cfblk26/1
  cfblk26/1 -> cfblk14/1
  cfblk12/1 -> cfblk27/1
  cfblk27/1 -> cfblk18/2(cfblk9)
  cfblk6/1 -> cfblk28/1
  cfblk28/1 -> cfblk17/1(cfblk1)
  cfblk11/1 -> cfblk29/1
  cfblk29/1 -> cfblk15/1
  cfblk13/1 -> cfblk30/1
  cfblk30/1 -> cfblk24/1
  cfblk21/1(cfblk2) -> cfblk31/1
  cfblk31/1 -> cfblk13/1
  cfblk21/2(cfblk16) -> cfblk32/1
  cfblk32/1 -> cfblk13/2

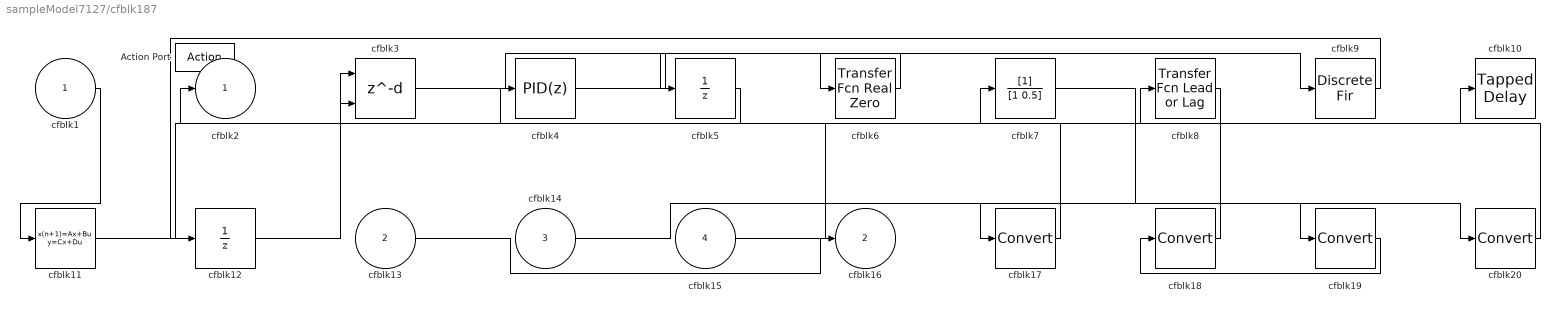
== system sampleModel7127/cfblk187 ==
  cfblk1 : Inport
  cfblk13 : Inport  Port=2
  cfblk14 : Inport  Port=3
  cfblk15 : Inport  Port=4
  Action Port : ActionPort  ActionType=then
  cfblk10 : simulink/Discrete/Tapped Delay  vinit=0.0  samptime=-1  NumDelays=1  DelayOrder=Oldest  includeCurrent=off
  cfblk11 : DiscreteStateSpace  SampleTime=-1
  cfblk12 : UnitDelay  SampleTime=-1
  cfblk{17..20} (4 alike) : DataTypeConversion
  cfblk3 : Delay  DelayLengthSource=Input port
      settings: InputPortMap=u0,p1
  cfblk4 : simulink/Continuous/PID Controller  Controller=PID  TimeDomain=Discrete-time  SampleTime=-1  IntegratorMethod=Forward Euler  FilterMethod=Forward Euler  Form=Parallel  UseFilter=on  ControllerParametersSource=internal  P=1  I=1  D=0  N=100  InitialConditionSource=internal  InitialConditionForIntegrator=0  InitialConditionForFilter=0  ExternalReset=none  LimitOutput=off  UpperSaturationLimit=inf  LowerSaturationLimit=-inf  LinearizeAsGain=off  AntiWindupMode=none  Kb=1  TrackingMode=off  Kt=1  PParamMin=[]  PParamMax=[]  IParamMin=[]  IParamMax=[]  DParamMin=[]  DParamMax=[]  NParamMin=[]  NParamMax=[]  KbParamMin=[]  KbParamMax=[]  KtParamMin=[]  KtParamMax=[]  POutMin=[]  POutMax=[]  IOutMin=[]  IOutMax=[]  DOutMin=[]  DOutMax=[]  NOutMin=[]  NOutMax=[]  KbOutMin=[]  KbOutMax=[]  KtOutMin=[]  KtOutMax=[]  IntegratorOutMin=[]  IntegratorOutMax=[]  FilterOutMin=[]  FilterOutMax=[]  SumOutMin=[]  SumOutMax=[]  SumI1OutMin=[]  SumI1OutMax=[]  SumI2OutMin=[]  SumI2OutMax=[]  SumI3OutMin=[]  SumI3OutMax=[]  SumDOutMin=[]  SumDOutMax=[]  SaturationOutMin=[]  SaturationOutMax=[]  IntegratorContinuousStateAttributes=''  IntegratorStateMustResolveToSignalObject=off  IntegratorRTWStateStorageClass=Auto  FilterContinuousStateAttributes=''  FilterStateMustResolveToSignalObject=off  FilterRTWStateStorageClass=Auto  DifferentiatorICPrevScaledInput=0  DifferentiatorOutMin=[]  DifferentiatorOutMax=[]  InitialConditionSetting=State (most efficient)
  cfblk5 : UnitDelay  SampleTime=-1
  cfblk6 : simulink/Discrete/Transfer Fcn Real Zero  ZeroZ=0.75  ICPrevInput=0.0  DoSatur=off
      settings: SourceProductName=Simulink  SourceProductBaseCode=SL
  cfblk7 : DiscreteFilter
  cfblk8 : simulink/Discrete/Transfer Fcn Lead or Lag  PoleZ=0.95  ZeroZ=0.75  ICPrevOutput=0.0  ICPrevInput=0.0  DoSatur=off
      settings: SourceProductName=Simulink  SourceProductBaseCode=SL
  cfblk9 : DiscreteFir
  cfblk2 : Outport
  cfblk16 : Outport  Port=2
  wires:
  cfblk1/1 -> cfblk11/1
  cfblk5/1 -> cfblk2/1
  cfblk4/1 -> cfblk9/1
  cfblk3/1 -> cfblk6/1
  cfblk15/1 -> cfblk10/1
  cfblk9/1 -> cfblk12/1
  cfblk11/1 -> cfblk4/1
  cfblk13/1 -> cfblk16/1
  cfblk6/1 -> cfblk5/1
  cfblk12/1 -> cfblk3/1
  cfblk8/1 -> cfblk17/1
  cfblk17/1 -> cfblk3/2
  cfblk18/1 -> cfblk8/1
  cfblk7/1 -> cfblk19/1
  cfblk19/1 -> cfblk18/1
  cfblk14/1 -> cfblk20/1
  cfblk20/1 -> cfblk7/1

== system sampleModel7127/cfblk188 ==
  cfblk1 : Inport
  Action Port : ActionPort  ActionType=else
  cfblk10 : DiscreteTransferFcn
  cfblk3 : DiscreteFir
  cfblk4 : DiscreteTransferFcn
  cfblk5 : DiscreteIntegrator  InitialConditionSetting=State (most efficient)  SampleTime=-1  ICPrevOutput=DiscIntNeverNeededParam  ICPrevScaledInput=DiscIntNeverNeededParam
  cfblk6 : DiscreteFilter
  cfblk7 : DiscreteTransferFcn
  cfblk8 : simulink/Discrete/Transfer Fcn First Order  PoleZ=0.95  ICPrevOutput=0.0  DoSatur=off
      settings: SourceProductName=Simulink
  cfblk9 : simulink/Discrete/Tapped Delay  vinit=0.0  samptime=-1  NumDelays=1  DelayOrder=Oldest  includeCurrent=off
  cfblk2 : Outport
  cfblk11 : Outport  Port=2
  wires:
  cfblk4/1 -> cfblk7/1
  cfblk6/1 -> cfblk8/1
  cfblk8/1 -> cfblk5/1
  cfblk10/1 -> cfblk11/1
  cfblk1/1 -> cfblk9/1
  cfblk7/1 -> cfblk6/1
  cfblk5/1 -> cfblk2/1
  cfblk3/1 -> cfblk4/1, cfblk10/1
  cfblk9/1 -> cfblk3/1

== system sampleModel7127/cfblk189 ==
  cfblk1 : Inport
  cfblk7 : Inport  Port=2
  cfblk8 : Inport  Port=3
  Action Port : ActionPort  ActionType=then
  cfblk3 : Delay
  cfblk4 : simulink/Continuous/PID Controller  Controller=PID  TimeDomain=Discrete-time  SampleTime=-1  IntegratorMethod=Forward Euler  FilterMethod=Forward Euler  Form=Parallel  UseFilter=on  ControllerParametersSource=internal  P=1  I=1  D=0  N=100  InitialConditionSource=internal  InitialConditionForIntegrator=0  InitialConditionForFilter=0  ExternalReset=none  LimitOutput=off  UpperSaturationLimit=inf  LowerSaturationLimit=-inf  LinearizeAsGain=off  AntiWindupMode=none  Kb=1  TrackingMode=off  Kt=1  PParamMin=[]  PParamMax=[]  IParamMin=[]  IParamMax=[]  DParamMin=[]  DParamMax=[]  NParamMin=[]  NParamMax=[]  KbParamMin=[]  KbParamMax=[]  KtParamMin=[]  KtParamMax=[]  POutMin=[]  POutMax=[]  IOutMin=[]  IOutMax=[]  DOutMin=[]  DOutMax=[]  NOutMin=[]  NOutMax=[]  KbOutMin=[]  KbOutMax=[]  KtOutMin=[]  KtOutMax=[]  IntegratorOutMin=[]  IntegratorOutMax=[]  FilterOutMin=[]  FilterOutMax=[]  SumOutMin=[]  SumOutMax=[]  SumI1OutMin=[]  SumI1OutMax=[]  SumI2OutMin=[]  SumI2OutMax=[]  SumI3OutMin=[]  SumI3OutMax=[]  SumDOutMin=[]  SumDOutMax=[]  SaturationOutMin=[]  SaturationOutMax=[]  IntegratorContinuousStateAttributes=''  IntegratorStateMustResolveToSignalObject=off  IntegratorRTWStateStorageClass=Auto  FilterContinuousStateAttributes=''  FilterStateMustResolveToSignalObject=off  FilterRTWStateStorageClass=Auto  DifferentiatorICPrevScaledInput=0  DifferentiatorOutMin=[]  DifferentiatorOutMax=[]  InitialConditionSetting=State (most efficient)
  cfblk5 : DiscreteStateSpace  SampleTime=-1
  cfblk6 : simulink/Discrete/Tapped Delay  vinit=0.0  samptime=-1  NumDelays=1  DelayOrder=Oldest  includeCurrent=off
  cfblk2 : Outport
  wires:
  cfblk7/1 -> cfblk3/1
  cfblk8/1 -> cfblk5/1
  cfblk5/1 -> cfblk6/1
  cfblk3/1 -> cfblk4/1
  cfblk4/1 -> cfblk2/1

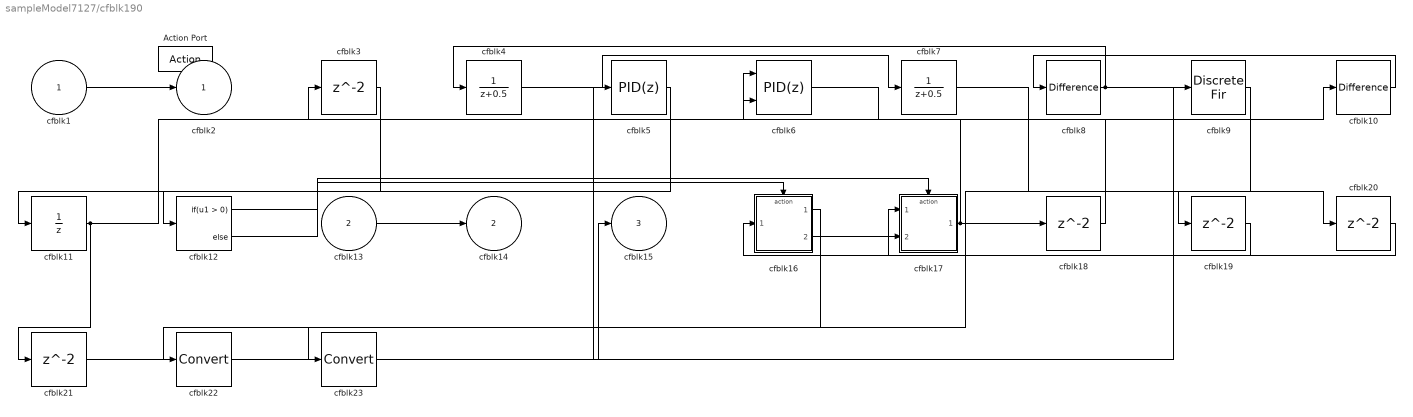
== system sampleModel7127/cfblk190 ==
  cfblk1 : Inport
  cfblk13 : Inport  Port=2
  Action Port : ActionPort  ActionType=else
  cfblk10 : simulink/Discrete/Difference  ICPrevInput=0.0  OutMin=[]  OutMax=[]  OutDataTypeStr=Inherit: Inherit via back propagation  OutDataType=fixdt(1, 16)  OutScaling=2^-10  DoSatur=off
  cfblk11 : UnitDelay  SampleTime=-1
  cfblk12 : If  SampleTime=1
  cfblk16 : Subsystem  TreatAsAtomicUnit=on
  cfblk17 : Subsystem  TreatAsAtomicUnit=on
  cfblk{3,18..21} (5 alike) : Delay
  cfblk22 : DataTypeConversion
  cfblk23 : DataTypeConversion
  cfblk4 : DiscreteTransferFcn
  cfblk5 : simulink/Continuous/PID Controller  Controller=PID  TimeDomain=Discrete-time  SampleTime=-1  IntegratorMethod=Forward Euler  FilterMethod=Forward Euler  Form=Parallel  UseFilter=on  ControllerParametersSource=internal  P=1  I=1  D=0  N=100  InitialConditionSource=internal  InitialConditionForIntegrator=0  InitialConditionForFilter=0  ExternalReset=none  LimitOutput=off  UpperSaturationLimit=inf  LowerSaturationLimit=-inf  LinearizeAsGain=off  AntiWindupMode=none  Kb=1  TrackingMode=off  Kt=1  PParamMin=[]  PParamMax=[]  IParamMin=[]  IParamMax=[]  DParamMin=[]  DParamMax=[]  NParamMin=[]  NParamMax=[]  KbParamMin=[]  KbParamMax=[]  KtParamMin=[]  KtParamMax=[]  POutMin=[]  POutMax=[]  IOutMin=[]  IOutMax=[]  DOutMin=[]  DOutMax=[]  NOutMin=[]  NOutMax=[]  KbOutMin=[]  KbOutMax=[]  KtOutMin=[]  KtOutMax=[]  IntegratorOutMin=[]  IntegratorOutMax=[]  FilterOutMin=[]  FilterOutMax=[]  SumOutMin=[]  SumOutMax=[]  SumI1OutMin=[]  SumI1OutMax=[]  SumI2OutMin=[]  SumI2OutMax=[]  SumI3OutMin=[]  SumI3OutMax=[]  SumDOutMin=[]  SumDOutMax=[]  SaturationOutMin=[]  SaturationOutMax=[]  IntegratorContinuousStateAttributes=''  IntegratorStateMustResolveToSignalObject=off  IntegratorRTWStateStorageClass=Auto  FilterContinuousStateAttributes=''  FilterStateMustResolveToSignalObject=off  FilterRTWStateStorageClass=Auto  DifferentiatorICPrevScaledInput=0  DifferentiatorOutMin=[]  DifferentiatorOutMax=[]  InitialConditionSetting=State (most efficient)
  cfblk6 : simulink/Continuous/PID Controller (2DOF)  Controller=PID  TimeDomain=Discrete-time  SampleTime=-1  IntegratorMethod=Forward Euler  FilterMethod=Forward Euler  Form=Parallel  UseFilter=on  ControllerParametersSource=internal  P=1  I=1  D=0  N=100  b=1  c=1  InitialConditionSource=internal  InitialConditionForIntegrator=0  InitialConditionForFilter=0  ExternalReset=none  LimitOutput=off  UpperSaturationLimit=inf  LowerSaturationLimit=-inf  LinearizeAsGain=off  AntiWindupMode=none  Kb=1  TrackingMode=off  Kt=1  PParamMin=[]  PParamMax=[]  IParamMin=[]  IParamMax=[]  DParamMin=[]  DParamMax=[]  NParamMin=[]  NParamMax=[]  bParamMin=[]  bParamMax=[]  cParamMin=[]  cParamMax=[]  KbParamMin=[]  KbParamMax=[]  KtParamMin=[]  KtParamMax=[]  POutMin=[]  POutMax=[]  IOutMin=[]  IOutMax=[]  DOutMin=[]  DOutMax=[]  NOutMin=[]  NOutMax=[]  bOutMin=[]  bOutMax=[]  cOutMin=[]  cOutMax=[]  KbOutMin=[]  KbOutMax=[]  KtOutMin=[]  KtOutMax=[]  IntegratorOutMin=[]  IntegratorOutMax=[]  FilterOutMin=[]  FilterOutMax=[]  SumOutMin=[]  SumOutMax=[]  Sum1OutMin=[]  Sum1OutMax=[]  Sum2OutMin=[]  Sum2OutMax=[]  Sum3OutMin=[]  Sum3OutMax=[]  SumI1OutMin=[]  SumI1OutMax=[]  SumI2OutMin=[]  SumI2OutMax=[]  SumI3OutMin=[]  SumI3OutMax=[]  SumDOutMin=[]  SumDOutMax=[]  SaturationOutMin=[]  SaturationOutMax=[]  IntegratorContinuousStateAttributes=''  IntegratorStateMustResolveToSignalObject=off  IntegratorRTWStateStorageClass=Auto  FilterContinuousStateAttributes=''  FilterStateMustResolveToSignalObject=off  FilterRTWStateStorageClass=Auto  DifferentiatorICPrevScaledInput=0  DifferentiatorOutMin=[]  DifferentiatorOutMax=[]  InitialConditionSetting=State (most efficient)
  cfblk7 : DiscreteTransferFcn
  cfblk8 : simulink/Discrete/Difference  ICPrevInput=0.0  OutMin=[]  OutMax=[]  OutDataTypeStr=Inherit: Inherit via back propagation  OutDataType=fixdt(1, 16)  OutScaling=2^-10  DoSatur=off
  cfblk9 : DiscreteFir
  cfblk2 : Outport
  cfblk14 : Outport  Port=2
  cfblk15 : Outport  Port=3
  wires:
  cfblk4/1 -> cfblk7/1
  cfblk13/1 -> cfblk14/1
  cfblk3/1 -> cfblk12/1
  cfblk1/1 -> cfblk2/1
  cfblk6/1 -> cfblk10/1
  cfblk17/1(cfblk2) -> cfblk6/1, cfblk18/1
  cfblk8/1 -> cfblk4/1, cfblk20/1
  cfblk10/1 -> cfblk8/1
  cfblk11/1 -> cfblk6/2, cfblk21/1
  cfblk16/2(cfblk7) -> cfblk17/1(cfblk1)
  cfblk5/1 -> cfblk11/1
  cfblk12/1 -> cfblk16/Action
  cfblk12/2 -> cfblk17/Action
  cfblk18/1 -> cfblk3/1
  cfblk7/1 -> cfblk19/1
  cfblk19/1 -> cfblk16/1(cfblk1)
  cfblk20/1 -> cfblk17/2(cfblk9)
  cfblk21/1 -> cfblk5/1
  cfblk9/1 -> cfblk22/1
  cfblk22/1 -> cfblk15/1
  cfblk16/1(cfblk2) -> cfblk23/1
  cfblk23/1 -> cfblk9/1

== system sampleModel7127/cfblk191 ==
  cfblk1 : Inport
  Action Port : ActionPort  ActionType=then
  cfblk10 : DiscreteFir
  cfblk11 : simulink/Continuous/PID Controller  Controller=PID  TimeDomain=Discrete-time  SampleTime=-1  IntegratorMethod=Forward Euler  FilterMethod=Forward Euler  Form=Parallel  UseFilter=on  ControllerParametersSource=internal  P=1  I=1  D=0  N=100  InitialConditionSource=internal  InitialConditionForIntegrator=0  InitialConditionForFilter=0  ExternalReset=none  LimitOutput=off  UpperSaturationLimit=inf  LowerSaturationLimit=-inf  LinearizeAsGain=off  AntiWindupMode=none  Kb=1  TrackingMode=off  Kt=1  PParamMin=[]  PParamMax=[]  IParamMin=[]  IParamMax=[]  DParamMin=[]  DParamMax=[]  NParamMin=[]  NParamMax=[]  KbParamMin=[]  KbParamMax=[]  KtParamMin=[]  KtParamMax=[]  POutMin=[]  POutMax=[]  IOutMin=[]  IOutMax=[]  DOutMin=[]  DOutMax=[]  NOutMin=[]  NOutMax=[]  KbOutMin=[]  KbOutMax=[]  KtOutMin=[]  KtOutMax=[]  IntegratorOutMin=[]  IntegratorOutMax=[]  FilterOutMin=[]  FilterOutMax=[]  SumOutMin=[]  SumOutMax=[]  SumI1OutMin=[]  SumI1OutMax=[]  SumI2OutMin=[]  SumI2OutMax=[]  SumI3OutMin=[]  SumI3OutMax=[]  SumDOutMin=[]  SumDOutMax=[]  SaturationOutMin=[]  SaturationOutMax=[]  IntegratorContinuousStateAttributes=''  IntegratorStateMustResolveToSignalObject=off  IntegratorRTWStateStorageClass=Auto  FilterContinuousStateAttributes=''  FilterStateMustResolveToSignalObject=off  FilterRTWStateStorageClass=Auto  DifferentiatorICPrevScaledInput=0  DifferentiatorOutMin=[]  DifferentiatorOutMax=[]  InitialConditionSetting=State (most efficient)
  cfblk12 : simulink/Continuous/PID Controller  Controller=PID  TimeDomain=Discrete-time  SampleTime=-1  IntegratorMethod=Forward Euler  FilterMethod=Forward Euler  Form=Parallel  UseFilter=on  ControllerParametersSource=internal  P=1  I=1  D=0  N=100  InitialConditionSource=internal  InitialConditionForIntegrator=0  InitialConditionForFilter=0  ExternalReset=none  LimitOutput=off  UpperSaturationLimit=inf  LowerSaturationLimit=-inf  LinearizeAsGain=off  AntiWindupMode=none  Kb=1  TrackingMode=off  Kt=1  PParamMin=[]  PParamMax=[]  IParamMin=[]  IParamMax=[]  DParamMin=[]  DParamMax=[]  NParamMin=[]  NParamMax=[]  KbParamMin=[]  KbParamMax=[]  KtParamMin=[]  KtParamMax=[]  POutMin=[]  POutMax=[]  IOutMin=[]  IOutMax=[]  DOutMin=[]  DOutMax=[]  NOutMin=[]  NOutMax=[]  KbOutMin=[]  KbOutMax=[]  KtOutMin=[]  KtOutMax=[]  IntegratorOutMin=[]  IntegratorOutMax=[]  FilterOutMin=[]  FilterOutMax=[]  SumOutMin=[]  SumOutMax=[]  SumI1OutMin=[]  SumI1OutMax=[]  SumI2OutMin=[]  SumI2OutMax=[]  SumI3OutMin=[]  SumI3OutMax=[]  SumDOutMin=[]  SumDOutMax=[]  SaturationOutMin=[]  SaturationOutMax=[]  IntegratorContinuousStateAttributes=''  IntegratorStateMustResolveToSignalObject=off  IntegratorRTWStateStorageClass=Auto  FilterContinuousStateAttributes=''  FilterStateMustResolveToSignalObject=off  FilterRTWStateStorageClass=Auto  DifferentiatorICPrevScaledInput=0  DifferentiatorOutMin=[]  DifferentiatorOutMax=[]  InitialConditionSetting=State (most efficient)
  cfblk13 : simulink/Discrete/Difference  ICPrevInput=0.0  OutMin=[]  OutMax=[]  OutDataTypeStr=Inherit: Inherit via back propagation  OutDataType=fixdt(1, 16)  OutScaling=2^-10  DoSatur=off
  cfblk14 : Delay
  cfblk15 : Delay
  cfblk3 : simulink/Discrete/Transfer Fcn First Order  PoleZ=0.95  ICPrevOutput=0.0  DoSatur=off
      settings: SourceProductName=Simulink
  cfblk4 : DiscreteZeroPole  Poles=[0 0.5]  Gain=1  SampleTime=-1
  cfblk5 : DiscreteTransferFcn
  cfblk6 : simulink/Continuous/PID Controller  Controller=PID  TimeDomain=Discrete-time  SampleTime=-1  IntegratorMethod=Forward Euler  FilterMethod=Forward Euler  Form=Parallel  UseFilter=on  ControllerParametersSource=internal  P=1  I=1  D=0  N=100  InitialConditionSource=internal  InitialConditionForIntegrator=0  InitialConditionForFilter=0  ExternalReset=none  LimitOutput=off  UpperSaturationLimit=inf  LowerSaturationLimit=-inf  LinearizeAsGain=off  AntiWindupMode=none  Kb=1  TrackingMode=off  Kt=1  PParamMin=[]  PParamMax=[]  IParamMin=[]  IParamMax=[]  DParamMin=[]  DParamMax=[]  NParamMin=[]  NParamMax=[]  KbParamMin=[]  KbParamMax=[]  KtParamMin=[]  KtParamMax=[]  POutMin=[]  POutMax=[]  IOutMin=[]  IOutMax=[]  DOutMin=[]  DOutMax=[]  NOutMin=[]  NOutMax=[]  KbOutMin=[]  KbOutMax=[]  KtOutMin=[]  KtOutMax=[]  IntegratorOutMin=[]  IntegratorOutMax=[]  FilterOutMin=[]  FilterOutMax=[]  SumOutMin=[]  SumOutMax=[]  SumI1OutMin=[]  SumI1OutMax=[]  SumI2OutMin=[]  SumI2OutMax=[]  SumI3OutMin=[]  SumI3OutMax=[]  SumDOutMin=[]  SumDOutMax=[]  SaturationOutMin=[]  SaturationOutMax=[]  IntegratorContinuousStateAttributes=''  IntegratorStateMustResolveToSignalObject=off  IntegratorRTWStateStorageClass=Auto  FilterContinuousStateAttributes=''  FilterStateMustResolveToSignalObject=off  FilterRTWStateStorageClass=Auto  DifferentiatorICPrevScaledInput=0  DifferentiatorOutMin=[]  DifferentiatorOutMax=[]  InitialConditionSetting=State (most efficient)
  cfblk7 : simulink/Discrete/Transfer Fcn Real Zero  ZeroZ=0.75  ICPrevInput=0.0  DoSatur=off
      settings: SourceProductName=Simulink  SourceProductBaseCode=SL
  cfblk8 : simulink/Discrete/Tapped Delay  vinit=0.0  samptime=-1  NumDelays=1  DelayOrder=Oldest  includeCurrent=off
  cfblk9 : simulink/Discrete/Difference  ICPrevInput=0.0  OutMin=[]  OutMax=[]  OutDataTypeStr=Inherit: Inherit via back propagation  OutDataType=fixdt(1, 16)  OutScaling=2^-10  DoSatur=off
  cfblk2 : Outport
  wires:
  cfblk3/1 -> cfblk12/1
  cfblk8/1 -> cfblk13/1
  cfblk13/1 -> cfblk5/1
  cfblk11/1 -> cfblk10/1
  cfblk4/1 -> cfblk9/1
  cfblk12/1 -> cfblk8/1
  cfblk5/1 -> cfblk6/1
  cfblk6/1 -> cfblk7/1
  cfblk1/1 -> cfblk2/1
  cfblk7/1 -> cfblk11/1
  cfblk10/1 -> cfblk14/1
  cfblk14/1 -> cfblk3/1
  cfblk9/1 -> cfblk15/1
  cfblk15/1 -> cfblk4/1

== system sampleModel7127/cfblk192 ==
  cfblk1 : Inport
  cfblk8 : Inport  Port=2
  Action Port : ActionPort  ActionType=else
  cfblk3 : DiscreteStateSpace  SampleTime=-1
  cfblk4 : simulink/Discrete/Transfer Fcn Real Zero  ZeroZ=0.75  ICPrevInput=0.0  DoSatur=off
      settings: SourceProductName=Simulink  SourceProductBaseCode=SL
  cfblk5 : simulink/Discrete/Difference  ICPrevInput=0.0  OutMin=[]  OutMax=[]  OutDataTypeStr=Inherit: Inherit via back propagation  OutDataType=fixdt(1, 16)  OutScaling=2^-10  DoSatur=off
  cfblk6 : DiscreteZeroPole  Poles=[0 0.5]  Gain=1  SampleTime=-1
  cfblk7 : simulink/Continuous/PID Controller (2DOF)  Controller=PID  TimeDomain=Discrete-time  SampleTime=-1  IntegratorMethod=Forward Euler  FilterMethod=Forward Euler  Form=Parallel  UseFilter=on  ControllerParametersSource=internal  P=1  I=1  D=0  N=100  b=1  c=1  InitialConditionSource=internal  InitialConditionForIntegrator=0  InitialConditionForFilter=0  ExternalReset=none  LimitOutput=off  UpperSaturationLimit=inf  LowerSaturationLimit=-inf  LinearizeAsGain=off  AntiWindupMode=none  Kb=1  TrackingMode=off  Kt=1  PParamMin=[]  PParamMax=[]  IParamMin=[]  IParamMax=[]  DParamMin=[]  DParamMax=[]  NParamMin=[]  NParamMax=[]  bParamMin=[]  bParamMax=[]  cParamMin=[]  cParamMax=[]  KbParamMin=[]  KbParamMax=[]  KtParamMin=[]  KtParamMax=[]  POutMin=[]  POutMax=[]  IOutMin=[]  IOutMax=[]  DOutMin=[]  DOutMax=[]  NOutMin=[]  NOutMax=[]  bOutMin=[]  bOutMax=[]  cOutMin=[]  cOutMax=[]  KbOutMin=[]  KbOutMax=[]  KtOutMin=[]  KtOutMax=[]  IntegratorOutMin=[]  IntegratorOutMax=[]  FilterOutMin=[]  FilterOutMax=[]  SumOutMin=[]  SumOutMax=[]  Sum1OutMin=[]  Sum1OutMax=[]  Sum2OutMin=[]  Sum2OutMax=[]  Sum3OutMin=[]  Sum3OutMax=[]  SumI1OutMin=[]  SumI1OutMax=[]  SumI2OutMin=[]  SumI2OutMax=[]  SumI3OutMin=[]  SumI3OutMax=[]  SumDOutMin=[]  SumDOutMax=[]  SaturationOutMin=[]  SaturationOutMax=[]  IntegratorContinuousStateAttributes=''  IntegratorStateMustResolveToSignalObject=off  IntegratorRTWStateStorageClass=Auto  FilterContinuousStateAttributes=''  FilterStateMustResolveToSignalObject=off  FilterRTWStateStorageClass=Auto  DifferentiatorICPrevScaledInput=0  DifferentiatorOutMin=[]  DifferentiatorOutMax=[]  InitialConditionSetting=State (most efficient)
  cfblk9 : Delay
  cfblk2 : Outport
  wires:
  cfblk8/1 -> cfblk7/1
  cfblk7/1 -> cfblk5/1
  cfblk5/1 -> cfblk4/1
  cfblk1/1 -> cfblk2/1
  cfblk4/1 -> cfblk6/1
  cfblk3/1 -> cfblk7/2
  cfblk6/1 -> cfblk9/1
  cfblk9/1 -> cfblk3/1
